simulink library "inputs_lib"  (R2020a)
settings: Solver=VariableStepAuto  StartTime=0.0  StopTime=10.0  RelTol=1e-3
libraries: SignalEditorBlockLib x1
settings Model: Creator=promero  LastModifiedBy=promero

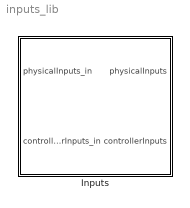
== system inputs_lib ==
  Inputs : Subsystem  Variant=on  VariantControlMode=Label  VariantControl=Choice  LabelModeActiveChoice=dashboardInput

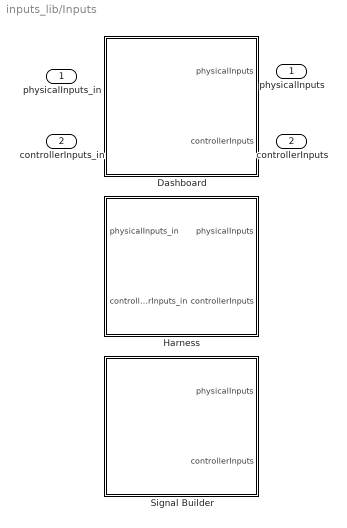
== system inputs_lib/Inputs ==
  physicalInputs_in : Inport  OutDataTypeStr=Bus: physicalInputs
  controllerInputs_in : Inport  Port=2  OutDataTypeStr=Bus: controllerInputs
  Dashboard : Subsystem  VariantControl=dashboardInput
  Harness : Subsystem  VariantControl=harnessInput
  Signal Builder : Subsystem  VariantControl=sigBuilderInput
  physicalInputs : Outport  OutDataTypeStr=Bus: physicalInputs
  controllerInputs : Outport  Port=2  OutDataTypeStr=Bus: controllerInputs

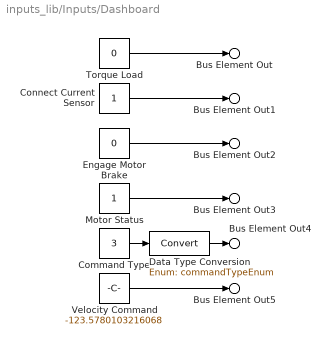
== system inputs_lib/Inputs/Dashboard ==
  Command Type : Constant  Value=3  OutDataTypeStr=uint8
  Connect Current Sensor : Constant  OutDataTypeStr=boolean
  Data Type Conversion : DataTypeConversion  OutDataTypeStr=Enum: commandTypeEnum
  Engage Motor Brake : Constant  Value=0  OutDataTypeStr=boolean
  Motor Status : Constant  OutDataTypeStr=boolean
  Torque Load : Constant  Value=0  OutDataTypeStr=Inherit: Inherit via back propagation
  Velocity Command : Constant  Value=-123.5780103216068  OutDataTypeStr=Inherit: Inherit via back propagation
  Bus Element Out : Outport  PortName=physicalInputs  Element=torqueLoad
  Bus Element Out1 : Outport  PortName=physicalInputs  Element=connectCurrentSensor
  Bus Element Out2 : Outport  PortName=physicalInputs  Element=motorBrake
  Bus Element Out3 : Outport  Port=2  PortName=controllerInputs  Element=motorOn
  Bus Element Out4 : Outport  Port=2  PortName=controllerInputs  Element=commandType
  Bus Element Out5 : Outport  Port=2  PortName=controllerInputs  Element=velocityCommand
  wires:
  Motor Status/1 -> Bus Element Out3/1
  Command Type/1 -> Data Type Conversion/1
  Velocity Command/1 -> Bus Element Out5/1
  Torque Load/1 -> Bus Element Out/1
  Connect Current Sensor/1 -> Bus Element Out1/1
  Data Type Conversion/1 -> Bus Element Out4/1
  Engage Motor Brake/1 -> Bus Element Out2/1

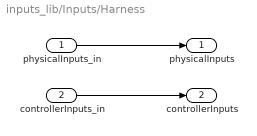
== system inputs_lib/Inputs/Harness ==
  physicalInputs_in : Inport  OutDataTypeStr=Bus: physicalInputs
  controllerInputs_in : Inport  Port=2  OutDataTypeStr=Bus: controllerInputs
  physicalInputs : Outport  OutDataTypeStr=Bus: physicalInputs
  controllerInputs : Outport  Port=2  OutDataTypeStr=Bus: controllerInputs
  wires:
  controllerInputs_in/1 -> controllerInputs/1
  physicalInputs_in/1 -> physicalInputs/1

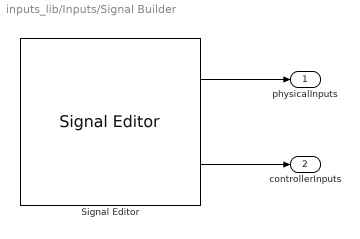
== system inputs_lib/Inputs/Signal Builder ==
  Signal Editor : SignalEditorBlockLib/Signal Editor  FileName=systemInputs.mat  ActiveScenario=doubleStepPosNegClosedLoop  ActiveSignal=controlInputs  IsBus=on  OutputBusObjectStr=Bus: controllerInputs  SampleTime=-1  Interpolate=off  ZeroCross=off  OutputAfterFinalValue=Holding final value  Unit=inherit  PreserveSignalName=on
  physicalInputs : Outport  OutDataTypeStr=Bus: physicalInputs
  controllerInputs : Outport  Port=2  OutDataTypeStr=Bus: controllerInputs
  wires:
  Signal Editor/2 -> controllerInputs/1
  Signal Editor/1 -> physicalInputs/1
